simulink model "Wiper_Manual"  (R2020b)
settings: Solver=VariableStepAuto  StartTime=0.0  StopTime=Inf  RelTol=1e-3
settings Model: Creator=99003778  LastModifiedBy=99003778

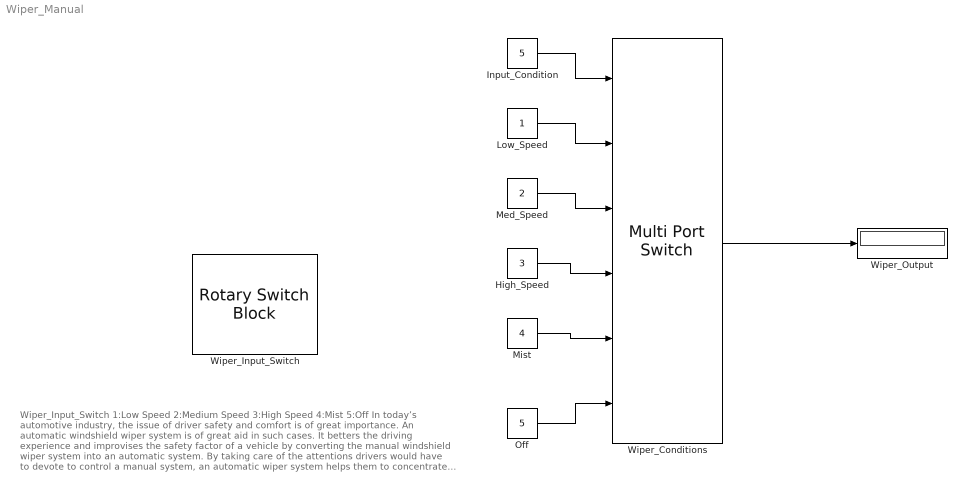
== system Wiper_Manual ==
  note: Wiper_Input_Switch
      | 1:Low Speed
      | 2:Medium Speed
      | 3:High Speed
      | 4:Mist
      | 5:Off
      | In today’s automotive industry, the issue of driver safety and comfort is of great importance. An automatic windshield wiper system is of great aid in such cases. It betters the driving experience and improvises the safety factor of a vehicle by converting the manual windshield wiper system into an automatic system. By taking care of the attentions drivers would have to devote to control a manual system, an automatic wiper system helps them to concentrate more on driving safely. Although, few automated windshield wiper systems are available in the automotive market, they are very costly and not very effective.
  High_Speed : Constant  Value=3
  Input_Condition : Constant  Value=5
  Low_Speed : Constant
  Med_Speed : Constant  Value=2
  Mist : Constant  Value=4
  Off : Constant  Value=5
  Wiper_Conditions : MultiPortSwitch  Inputs=5
  Wiper_Input_Switch : RotarySwitchBlock
      settings: Values={{'Off', 'Low', 'Medium', 'High', 'Mist'}, [5 1 2 3 4]}
  Wiper_Output : Display
  wires:
  Wiper_Conditions/1 -> Wiper_Output/1
  Input_Condition/1 -> Wiper_Conditions/1
  Low_Speed/1 -> Wiper_Conditions/2
  Med_Speed/1 -> Wiper_Conditions/3
  High_Speed/1 -> Wiper_Conditions/4
  Mist/1 -> Wiper_Conditions/5
  Off/1 -> Wiper_Conditions/6
